simulink model "gm_rmsNormalization"  (R2025a)
settings: Solver=FixedStepDiscrete  StartTime=0.0  StopTime=simStopTime  FixedStep=1  RelTol=1e-3
libraries: simulink x23
(part 3 of 3)

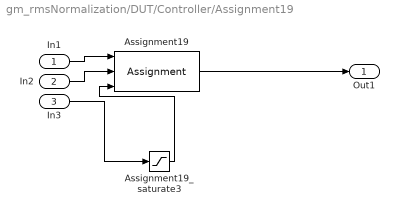
== system gm_rmsNormalization/DUT/Controller/Assignment19 ==
  In1 : Inport
  In2 : Inport  Port=2
  In3 : Inport  Port=3
  Assignment19 : Assignment  IndexOptions=Index vector (port)  Indices=double(-1)  OutputSizes=double(0)
  Assignment19_saturate3 : Saturate  UpperLimit=1536  LowerLimit=1
  Out1 : Outport
  wires:
  In3/1 -> Assignment19_saturate3/1
  Assignment19_saturate3/1 -> Assignment19/3
  In1/1 -> Assignment19/1
  In2/1 -> Assignment19/2
  Assignment19/1 -> Out1/1

== system gm_rmsNormalization/DUT/Controller/Assignment20 ==
  In1 : Inport
  In2 : Inport  Port=2
  In3 : Inport  Port=3
  Assignment20 : Assignment  IndexOptions=Index vector (port)  Indices=double(-1)  OutputSizes=double(0)
  Assignment20_saturate3 : Saturate  UpperLimit=1536  LowerLimit=1
  Out1 : Outport
  wires:
  In3/1 -> Assignment20_saturate3/1
  Assignment20_saturate3/1 -> Assignment20/3
  In1/1 -> Assignment20/1
  In2/1 -> Assignment20/2
  Assignment20/1 -> Out1/1

== system gm_rmsNormalization/DUT/Controller/Assignment21 ==
  In1 : Inport
  In2 : Inport  Port=2
  In3 : Inport  Port=3
  Assignment21 : Assignment  IndexOptions=Index vector (port)  Indices=double(-1)  OutputSizes=double(0)
  Assignment21_saturate3 : Saturate  UpperLimit=1536  LowerLimit=1
  Out1 : Outport
  wires:
  In3/1 -> Assignment21_saturate3/1
  Assignment21_saturate3/1 -> Assignment21/3
  In1/1 -> Assignment21/1
  In2/1 -> Assignment21/2
  Assignment21/1 -> Out1/1

== system gm_rmsNormalization/DUT/Controller/Assignment22 ==
  In1 : Inport
  In2 : Inport  Port=2
  In3 : Inport  Port=3
  Assignment22 : Assignment  IndexOptions=Index vector (port)  Indices=double(-1)  OutputSizes=double(0)
  Assignment22_saturate3 : Saturate  UpperLimit=1536  LowerLimit=1
  Out1 : Outport
  wires:
  In3/1 -> Assignment22_saturate3/1
  Assignment22_saturate3/1 -> Assignment22/3
  In1/1 -> Assignment22/1
  In2/1 -> Assignment22/2
  Assignment22/1 -> Out1/1

== system gm_rmsNormalization/DUT/Controller/Assignment23 ==
  In1 : Inport
  In2 : Inport  Port=2
  In3 : Inport  Port=3
  Assignment23 : Assignment  IndexOptions=Index vector (port)  Indices=double(-1)  OutputSizes=double(0)
  Assignment23_saturate3 : Saturate  UpperLimit=1536  LowerLimit=1
  Out1 : Outport
  wires:
  In3/1 -> Assignment23_saturate3/1
  Assignment23_saturate3/1 -> Assignment23/3
  In1/1 -> Assignment23/1
  In2/1 -> Assignment23/2
  Assignment23/1 -> Out1/1

== system gm_rmsNormalization/DUT/Controller/Assignment24 ==
  In1 : Inport
  In2 : Inport  Port=2
  In3 : Inport  Port=3
  Assignment24 : Assignment  IndexOptions=Index vector (port)  Indices=double(-1)  OutputSizes=double(0)
  Assignment24_saturate3 : Saturate  UpperLimit=1536  LowerLimit=1
  Out1 : Outport
  wires:
  In3/1 -> Assignment24_saturate3/1
  Assignment24_saturate3/1 -> Assignment24/3
  In1/1 -> Assignment24/1
  In2/1 -> Assignment24/2
  Assignment24/1 -> Out1/1

== system gm_rmsNormalization/DUT/Controller/Assignment25 ==
  In1 : Inport
  In2 : Inport  Port=2
  In3 : Inport  Port=3
  Assignment25 : Assignment  IndexOptions=Index vector (port)  Indices=double(-1)  OutputSizes=double(0)
  Assignment25_saturate3 : Saturate  UpperLimit=1536  LowerLimit=1
  Out1 : Outport
  wires:
  In3/1 -> Assignment25_saturate3/1
  Assignment25_saturate3/1 -> Assignment25/3
  In1/1 -> Assignment25/1
  In2/1 -> Assignment25/2
  Assignment25/1 -> Out1/1

== system gm_rmsNormalization/DUT/Controller/Assignment26 ==
  In1 : Inport
  In2 : Inport  Port=2
  In3 : Inport  Port=3
  Assignment26 : Assignment  IndexOptions=Index vector (port)  Indices=double(-1)  OutputSizes=double(0)
  Assignment26_saturate3 : Saturate  UpperLimit=1536  LowerLimit=1
  Out1 : Outport
  wires:
  In3/1 -> Assignment26_saturate3/1
  Assignment26_saturate3/1 -> Assignment26/3
  In1/1 -> Assignment26/1
  In2/1 -> Assignment26/2
  Assignment26/1 -> Out1/1

== system gm_rmsNormalization/DUT/Controller/Assignment27 ==
  In1 : Inport
  In2 : Inport  Port=2
  In3 : Inport  Port=3
  Assignment27 : Assignment  IndexOptions=Index vector (port)  Indices=double(-1)  OutputSizes=double(0)
  Assignment27_saturate3 : Saturate  UpperLimit=1536  LowerLimit=1
  Out1 : Outport
  wires:
  In3/1 -> Assignment27_saturate3/1
  Assignment27_saturate3/1 -> Assignment27/3
  In1/1 -> Assignment27/1
  In2/1 -> Assignment27/2
  Assignment27/1 -> Out1/1

== system gm_rmsNormalization/DUT/Controller/Assignment28 ==
  In1 : Inport
  In2 : Inport  Port=2
  In3 : Inport  Port=3
  Assignment28 : Assignment  IndexOptions=Index vector (port)  Indices=double(-1)  OutputSizes=double(0)
  Assignment28_saturate3 : Saturate  UpperLimit=1536  LowerLimit=1
  Out1 : Outport
  wires:
  In3/1 -> Assignment28_saturate3/1
  Assignment28_saturate3/1 -> Assignment28/3
  In1/1 -> Assignment28/1
  In2/1 -> Assignment28/2
  Assignment28/1 -> Out1/1

== system gm_rmsNormalization/DUT/Controller/Assignment29 ==
  In1 : Inport
  In2 : Inport  Port=2
  In3 : Inport  Port=3
  Assignment29 : Assignment  IndexOptions=Index vector (port)  Indices=double(-1)  OutputSizes=double(0)
  Assignment29_saturate3 : Saturate  UpperLimit=1536  LowerLimit=1
  Out1 : Outport
  wires:
  In3/1 -> Assignment29_saturate3/1
  Assignment29_saturate3/1 -> Assignment29/3
  In1/1 -> Assignment29/1
  In2/1 -> Assignment29/2
  Assignment29/1 -> Out1/1

== system gm_rmsNormalization/DUT/Controller/Assignment30 ==
  In1 : Inport
  In2 : Inport  Port=2
  In3 : Inport  Port=3
  Assignment30 : Assignment  IndexOptions=Index vector (port)  Indices=double(-1)  OutputSizes=double(0)
  Assignment30_saturate3 : Saturate  UpperLimit=1536  LowerLimit=1
  Out1 : Outport
  wires:
  In3/1 -> Assignment30_saturate3/1
  Assignment30_saturate3/1 -> Assignment30/3
  In1/1 -> Assignment30/1
  In2/1 -> Assignment30/2
  Assignment30/1 -> Out1/1

== system gm_rmsNormalization/DUT/Controller/Assignment31 ==
  In1 : Inport
  In2 : Inport  Port=2
  In3 : Inport  Port=3
  Assignment31 : Assignment  IndexOptions=Index vector (port)  Indices=double(-1)  OutputSizes=double(0)
  Assignment31_saturate3 : Saturate  UpperLimit=1536  LowerLimit=1
  Out1 : Outport
  wires:
  In3/1 -> Assignment31_saturate3/1
  Assignment31_saturate3/1 -> Assignment31/3
  In1/1 -> Assignment31/1
  In2/1 -> Assignment31/2
  Assignment31/1 -> Out1/1

== system gm_rmsNormalization/DUT/Controller/Selector ==
  In1 : Inport
  In2 : Inport  Port=2
  Selector : Selector  InputPortWidth=1536  IndexOptions=Index vector (port)  Indices=double(-1)  OutputSizes=double(0)
  Selector_saturate2 : Saturate  UpperLimit=1536  LowerLimit=1
  Out1 : Outport
  wires:
  In2/1 -> Selector_saturate2/1
  Selector_saturate2/1 -> Selector/2
  In1/1 -> Selector/1
  Selector/1 -> Out1/1

== system gm_rmsNormalization/DUT/Controller/Selector1 ==
  In1 : Inport
  In2 : Inport  Port=2
  Selector1 : Selector  InputPortWidth=1536  IndexOptions=Index vector (port)  Indices=double(-1)  OutputSizes=double(0)
  Selector1_saturate2 : Saturate  UpperLimit=1536  LowerLimit=1
  Out1 : Outport
  wires:
  In2/1 -> Selector1_saturate2/1
  Selector1_saturate2/1 -> Selector1/2
  In1/1 -> Selector1/1
  Selector1/1 -> Out1/1

== system gm_rmsNormalization/DUT/Controller/Selector11 ==
  In1 : Inport
  In2 : Inport  Port=2
  Selector11 : Selector  InputPortWidth=1536  IndexOptions=Index vector (port)  Indices=double(-1)  OutputSizes=double(0)
  Selector11_saturate2 : Saturate  UpperLimit=1536  LowerLimit=1
  Out1 : Outport
  wires:
  In2/1 -> Selector11_saturate2/1
  Selector11_saturate2/1 -> Selector11/2
  In1/1 -> Selector11/1
  Selector11/1 -> Out1/1

== system gm_rmsNormalization/DUT/Controller/Selector12 ==
  In1 : Inport
  In2 : Inport  Port=2
  Selector12 : Selector  InputPortWidth=1536  IndexOptions=Index vector (port)  Indices=double(-1)  OutputSizes=double(0)
  Selector12_saturate2 : Saturate  UpperLimit=1536  LowerLimit=1
  Out1 : Outport
  wires:
  In2/1 -> Selector12_saturate2/1
  Selector12_saturate2/1 -> Selector12/2
  In1/1 -> Selector12/1
  Selector12/1 -> Out1/1

== system gm_rmsNormalization/DUT/Controller/Selector14 ==
  In1 : Inport
  In2 : Inport  Port=2
  Selector14 : Selector  InputPortWidth=1536  IndexOptions=Index vector (port)  Indices=double(-1)  OutputSizes=double(0)
  Selector14_saturate2 : Saturate  UpperLimit=1536  LowerLimit=1
  Out1 : Outport
  wires:
  In2/1 -> Selector14_saturate2/1
  Selector14_saturate2/1 -> Selector14/2
  In1/1 -> Selector14/1
  Selector14/1 -> Out1/1

== system gm_rmsNormalization/DUT/Controller/Selector15 ==
  In1 : Inport
  In2 : Inport  Port=2
  Selector15 : Selector  InputPortWidth=1536  IndexOptions=Index vector (port)  Indices=double(-1)  OutputSizes=double(0)
  Selector15_saturate2 : Saturate  UpperLimit=1536  LowerLimit=1
  Out1 : Outport
  wires:
  In2/1 -> Selector15_saturate2/1
  Selector15_saturate2/1 -> Selector15/2
  In1/1 -> Selector15/1
  Selector15/1 -> Out1/1

== system gm_rmsNormalization/DUT/Controller/Selector17 ==
  In1 : Inport
  In2 : Inport  Port=2
  Selector17 : Selector  InputPortWidth=1536  IndexOptions=Index vector (port)  Indices=double(-1)  OutputSizes=double(0)
  Selector17_saturate2 : Saturate  UpperLimit=1536  LowerLimit=1
  Out1 : Outport
  wires:
  In2/1 -> Selector17_saturate2/1
  Selector17_saturate2/1 -> Selector17/2
  In1/1 -> Selector17/1
  Selector17/1 -> Out1/1

== system gm_rmsNormalization/DUT/Controller/Selector18 ==
  In1 : Inport
  In2 : Inport  Port=2
  Selector18 : Selector  InputPortWidth=1536  IndexOptions=Index vector (port)  Indices=double(-1)  OutputSizes=double(0)
  Selector18_saturate2 : Saturate  UpperLimit=1536  LowerLimit=1
  Out1 : Outport
  wires:
  In2/1 -> Selector18_saturate2/1
  Selector18_saturate2/1 -> Selector18/2
  In1/1 -> Selector18/1
  Selector18/1 -> Out1/1

== system gm_rmsNormalization/DUT/Controller/Selector2 ==
  In1 : Inport
  In2 : Inport  Port=2
  Selector2 : Selector  InputPortWidth=1536  IndexOptions=Index vector (port)  Indices=double(-1)  OutputSizes=double(0)
  Selector2_saturate2 : Saturate  UpperLimit=1536  LowerLimit=1
  Out1 : Outport
  wires:
  In2/1 -> Selector2_saturate2/1
  Selector2_saturate2/1 -> Selector2/2
  In1/1 -> Selector2/1
  Selector2/1 -> Out1/1

== system gm_rmsNormalization/DUT/Controller/Selector20 ==
  In1 : Inport
  In2 : Inport  Port=2
  Selector20 : Selector  InputPortWidth=1536  IndexOptions=Index vector (port)  Indices=double(-1)  OutputSizes=double(0)
  Selector20_saturate2 : Saturate  UpperLimit=1536  LowerLimit=1
  Out1 : Outport
  wires:
  In2/1 -> Selector20_saturate2/1
  Selector20_saturate2/1 -> Selector20/2
  In1/1 -> Selector20/1
  Selector20/1 -> Out1/1

== system gm_rmsNormalization/DUT/Controller/Selector3 ==
  In1 : Inport
  In2 : Inport  Port=2
  Selector3 : Selector  InputPortWidth=1536  IndexOptions=Index vector (port)  Indices=double(-1)  OutputSizes=double(0)
  Selector3_saturate2 : Saturate  UpperLimit=1536  LowerLimit=1
  Out1 : Outport
  wires:
  In2/1 -> Selector3_saturate2/1
  Selector3_saturate2/1 -> Selector3/2
  In1/1 -> Selector3/1
  Selector3/1 -> Out1/1

== system gm_rmsNormalization/DUT/Controller/Selector4 ==
  In1 : Inport
  In2 : Inport  Port=2
  Selector4 : Selector  InputPortWidth=1536  IndexOptions=Index vector (port)  Indices=double(-1)  OutputSizes=double(0)
  Selector4_saturate2 : Saturate  UpperLimit=1536  LowerLimit=1
  Out1 : Outport
  wires:
  In2/1 -> Selector4_saturate2/1
  Selector4_saturate2/1 -> Selector4/2
  In1/1 -> Selector4/1
  Selector4/1 -> Out1/1

== system gm_rmsNormalization/DUT/Controller/Selector5 ==
  In1 : Inport
  In2 : Inport  Port=2
  Selector5 : Selector  InputPortWidth=1536  IndexOptions=Index vector (port)  Indices=double(-1)  OutputSizes=double(0)
  Selector5_saturate2 : Saturate  UpperLimit=1536  LowerLimit=1
  Out1 : Outport
  wires:
  In2/1 -> Selector5_saturate2/1
  Selector5_saturate2/1 -> Selector5/2
  In1/1 -> Selector5/1
  Selector5/1 -> Out1/1

== system gm_rmsNormalization/DUT/Controller/Selector6 ==
  In1 : Inport
  In2 : Inport  Port=2
  Selector6 : Selector  InputPortWidth=1536  IndexOptions=Index vector (port)  Indices=double(-1)  OutputSizes=double(0)
  Selector6_saturate2 : Saturate  UpperLimit=1536  LowerLimit=1
  Out1 : Outport
  wires:
  In2/1 -> Selector6_saturate2/1
  Selector6_saturate2/1 -> Selector6/2
  In1/1 -> Selector6/1
  Selector6/1 -> Out1/1

== system gm_rmsNormalization/DUT/Controller/Selector8 ==
  In1 : Inport
  In2 : Inport  Port=2
  Selector8 : Selector  InputPortWidth=1536  IndexOptions=Index vector (port)  Indices=double(-1)  OutputSizes=double(0)
  Selector8_saturate2 : Saturate  UpperLimit=1536  LowerLimit=1
  Out1 : Outport
  wires:
  In2/1 -> Selector8_saturate2/1
  Selector8_saturate2/1 -> Selector8/2
  In1/1 -> Selector8/1
  Selector8/1 -> Out1/1

== system gm_rmsNormalization/DUT/Controller/Selector9 ==
  In1 : Inport
  In2 : Inport  Port=2
  Selector9 : Selector  InputPortWidth=1536  IndexOptions=Index vector (port)  Indices=double(-1)  OutputSizes=double(0)
  Selector9_saturate2 : Saturate  UpperLimit=1536  LowerLimit=1
  Out1 : Outport
  wires:
  In2/1 -> Selector9_saturate2/1
  Selector9_saturate2/1 -> Selector9/2
  In1/1 -> Selector9/1
  Selector9/1 -> Out1/1

== system gm_rmsNormalization/DUT/Controller/adder33 ==
  In1 : Inport
  In2 : Inport  Port=2
  adder33 : Sum  OutDataTypeStr=single  SampleTime=1
  adder33_pd1 : Delay  DelayLength=11
  Out1 : Outport
  wires:
  In1/1 -> adder33/1
  In2/1 -> adder33/2
  adder33/1 -> adder33_pd1/1
  adder33_pd1/1 -> Out1/1

== system gm_rmsNormalization/DUT/LaneMultiply/ScaleGamma ==
  In1 : Inport
  In2 : Inport  Port=2
  ScaleGamma : Product  Inputs=**  OutDataTypeStr=single  SampleTime=1
  ScaleGamma_pd1 : Delay  DelayLength=8
  Out1 : Outport
  wires:
  In1/1 -> ScaleGamma/1
  In2/1 -> ScaleGamma/2
  ScaleGamma/1 -> ScaleGamma_pd1/1
  ScaleGamma_pd1/1 -> Out1/1

== system gm_rmsNormalization/DUT/LaneMultiply/ScaleMultiply ==
  In1 : Inport
  In2 : Inport  Port=2
  ScaleMultiply : Product  Inputs=**  OutDataTypeStr=single  SampleTime=1
  ScaleMultiply_pd1 : Delay  DelayLength=8
  Out1 : Outport
  wires:
  In1/1 -> ScaleMultiply/1
  In2/1 -> ScaleMultiply/2
  ScaleMultiply/1 -> ScaleMultiply_pd1/1
  ScaleMultiply_pd1/1 -> Out1/1

== system gm_rmsNormalization/DUT/LaneMultiply/WeightMultiply ==
  In1 : Inport
  In2 : Inport  Port=2
  WeightMultiply : Product  Inputs=**  OutDataTypeStr=single  SampleTime=1
  WeightMultiply_pd1 : Delay  DelayLength=8
  Out1 : Outport
  wires:
  In1/1 -> WeightMultiply/1
  In2/1 -> WeightMultiply/2
  WeightMultiply/1 -> WeightMultiply_pd1/1
  WeightMultiply_pd1/1 -> Out1/1

== system gm_rmsNormalization/DUT/ScalarRsqrt/Reciprocal ==
  In1 : Inport
  In2 : Inport  Port=2
  Reciprocal : Product  Inputs=*/  OutDataTypeStr=single  RndMeth=Zero  SaturateOnIntegerOverflow=on  SampleTime=1
  Reciprocal_pd1 : Delay  DelayLength=32
  Out1 : Outport
  wires:
  In1/1 -> Reciprocal/1
  In2/1 -> Reciprocal/2
  Reciprocal/1 -> Reciprocal_pd1/1
  Reciprocal_pd1/1 -> Out1/1

== system gm_rmsNormalization/DUT/ScalarRsqrt/Sqrt ==
  In1 : Inport
  Sqrt : Sqrt  SampleTime=1
  Sqrt_pd1 : Delay  DelayLength=28
  Out1 : Outport
  wires:
  In1/1 -> Sqrt/1
  Sqrt/1 -> Sqrt_pd1/1
  Sqrt_pd1/1 -> Out1/1

== system gm_rmsNormalization/DUT/SquareBeat/Square ==
  In1 : Inport
  In2 : Inport  Port=2
  Square : Product  Inputs=**  OutDataTypeStr=single  SampleTime=1
  Square_pd1 : Delay  DelayLength=8
  Out1 : Outport
  wires:
  In1/1 -> Square/1
  In2/1 -> Square/2
  Square/1 -> Square_pd1/1
  Square_pd1/1 -> Out1/1
